simulink model "Compensated_Controller"  (R2020b)
settings: Solver=VariableStepAuto  StartTime=0.0  StopTime=5  RelTol=1e-3
model workspace (MAT data in the model file):
  A = [0  1  0  0; 0  -0.363636363636  2.67272727273  0; 0  0  0  1; 0  -0.909090909091  31.1818181818  0]
  B = [0; 1.81818181818; 0; 4.54545454545]
  C = Simulink.Parameter
  C.Value = [1  0  0  0; 0  1  0  0; 0  0  1  0; 0  0  0  1]
  C.DataType = 'auto'
  C.Dimensions = [4 4]
  D = [0; 0; 0; 0]
  K = Simulink.Parameter
  K.Value = [-70.7107 -37.9361 105.5362 20.9251]
  K.DataType = 'auto'
  K.Dimensions = [1 4]
  Nbar = Simulink.Parameter
  Nbar.Value = -71
  Nbar.DataType = 'auto'
  Nbar.Dimensions = [1 1]
settings Model: Creator=Alvaro  LastModifiedBy=Alvaro

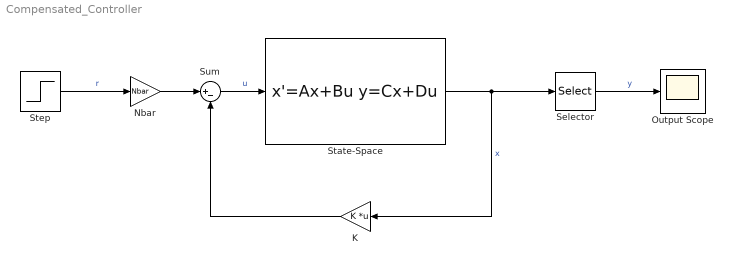
== system Compensated_Controller ==
  K : Gain  Gain=K  Multiplication=Matrix(K*u)
  Nbar : Gain  Gain=Nbar
  "Output Scope " : Scope
  Selector : Selector  InputPortWidth=4  IndexOptions=Index vector (dialog)  Indices=[1 3]  OutputSizes=1
  State-Space : StateSpace  A=A  B=B  C=C  D=D  InitialCondition=0  ContinuousStateAttributes={'cart_position', 'cart_velocity', 'pendulum_angle', 'pendulum_angle_rate'}
  Step : Step  Time=0.01  After=0.2  SampleTime=0.01
  Sum : Sum  Inputs=|+-
  wires:
  Nbar/1 -> Sum/1
  Step/1 -> Nbar/1  "r"
  State-Space/1 -> K/1, Selector/1  "x"
  Sum/1 -> State-Space/1  "u"
  Selector/1 -> "Output Scope "/1  "y"
  K/1 -> Sum/2
